simulink model "chaos_buck_CCM"  (R2021a)
settings: Solver=ode8  StartTime=0.0  StopTime=0.1  FixedStep=1e-6  RelTol=1e-3
model workspace (MAT data in the model file):
  C = Simulink.Parameter
  C.Value = [2.5e-05 2.51e-05 2.52e-05 2.53e-05 2.54e-05 2.55e-05 2.56e-05 2.57e-05 2.58e-05 2.59e-05 2.6e-05 2.61e-05 ... (351 elements, 1x351)]
  C.DataType = 'auto'
  C.Dimensions = [1 351]
  L = Simulink.Parameter
  L.Value = [0.01 0.0101 0.0102 0.0103 0.0104 0.0105 0.0106 0.0107 0.0108 0.0109 0.011 0.0111 0.0112 0.0113 0.0114 0.0115 0.0116 0.0117 0.0118 0.0119 0.012 0.0121 0.0122 0.0123 0.0124 0.0125 0.0126 0.0127 0.0128 0.0129 0.013 0.0131 0.0132 0.0133 0.0134 0.0135 0.0136 0.0137 0.0138 0.0139 0.014 0.0141 0.0142 0.0143 0.0144 0.0145 0.0146 0.0147 0.0148 0.0149 0.015 0.0151 0.0152 0.0153 0.0154 0.0155 0.0156 0.0157 0.0158 0.0159 0.016 0.0161 0.0162 0.0163 0.0164 0.0165 0.0166 0.0167 0.0168 0.0169 0.017 0.0171 0.0172 0.0173 0.0174 0.0175 0.0176 0.0177 0.0178 0.0179 0.018 0.0181 0.0182 0.0183 0.0184 0.0185 0.0186 0.0187 0.0188 0.0189 0.019 0.0191 0.0192 0.0193 0.0194 0.0195 0.0196 0.0197 0.0198 0.0199 0.02 0.0201 0.0202 0.0203 0.0204 0.0205 0.0206 0.0207 0.0208 0.0209 0.021 0.0211 0.0212 0.0213 0.0214 0.0215 0.0216 0.0217 0.0218 0.0219 0.022 0.0221 0.0222 0.0223 0.0224 0.0225 0.0226 0.0227 0.0228 0.0229 0.023 0.0231 0.0232 0.0233 0.0234 0.0235 0.0236 0.0237 0.0238 0.0239 0.024 0.0241 0.0242 0.0243 0.0244 0.0245 0.0246 0.0247 0.0248 0.0249 0.025]
  L.DataType = 'auto'
  L.Dimensions = [1 151]
  Vin = Simulink.Parameter
  Vin.Value = [20 20.1 20.2 20.3 20.4 20.5 20.6 20.7 20.8 20.9 21 21.1 21.2 21.3 21.4 21.5 21.6 21.7 21.8 21.9 22 22.1 22.2 22.3 22.4 22.5 22.6 22.7 22.8 22.9 23 23.1 23.2 23.3 23.4 23.5 23.6 23.7 23.8 23.9 24 24.1 24.2 24.3 24.4 24.5 24.6 24.7 24.8 24.9 25 25.1 25.2 25.3 25.4 25.5 25.6 25.7 25.8 25.9 26 26.1 26.2 26.3 26.4 26.5 26.6 26.7 26.8 26.9 27 27.1 27.2 27.3 27.4 27.5 27.6 27.7 27.8 27.9 28 28.1 28.2 28.3 28.4 28.5 28.6 28.7 28.8 28.9 29 29.1 29.2 29.3 29.4 29.5 29.6 29.7 29.8 29.9 30 30.1 30.2 30.3 30.4 30.5 30.6 30.7 30.8 30.9 31 31.1 31.2 31.3 31.4 31.5 31.6 31.7 31.8 31.9 32 32.1 32.2 32.3 32.4 32.5 32.6 32.7 32.8 32.9 33 33.1 33.2 33.3 33.4 33.5 33.6 33.7 33.8 33.9 34 34.1 34.2 34.3 34.4 34.5 34.6 34.7 34.8 34.9 35]
  Vin.DataType = 'auto'
  Vin.Dimensions = [1 151]
values from neighbouring files (symbols this model uses):
  Vin = 22    [CCM_iterative_mapping.m]    (also in DCM_iterative_mapping_bifur.m = 33)
libraries: simulink x1
settings Model: OrderedModelArguments=off  Creator=xiang zhang  LastModifiedBy=xiang zhang

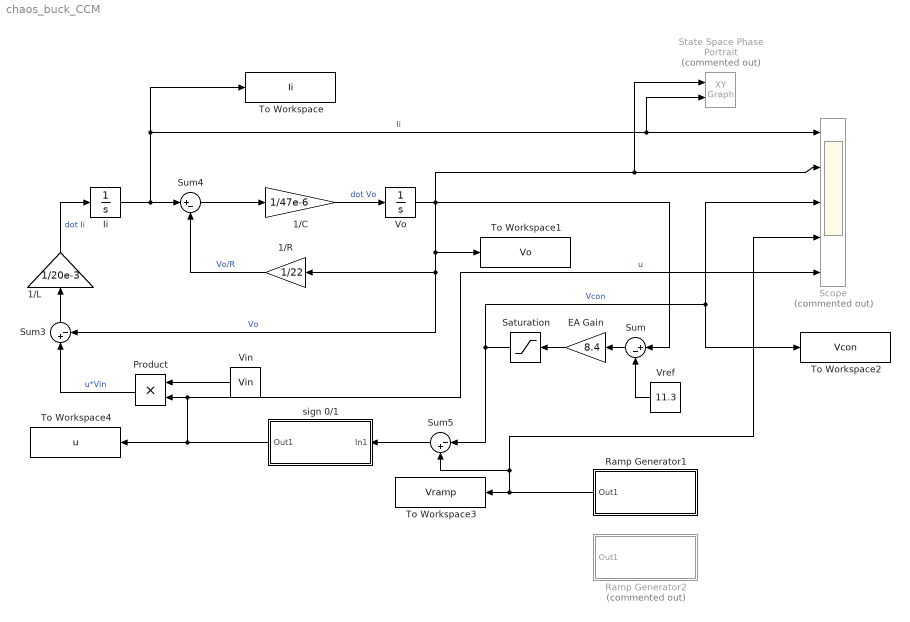
== system chaos_buck_CCM ==
  1/C : Gain  Gain=1/47e-6
  1/L : Gain  Gain=1/20e-3
  1/R : Gain  Gain=1/22
  EA Gain : Gain  Gain=8.4
  Ii : Integrator
  Product : Product
  Ramp Generator1 : Subsystem
  Ramp Generator2 : Subsystem  Commented=on
  Saturation : Saturate  UpperLimit=8.2  LowerLimit=3.8
  Scope : Scope  Commented=on  NumInputPorts=5
  State Space Phase Portrait : simulink/Sinks/XY Graph  Commented=on  xmin=10  xmax=14  ymin=-0.5  ymax=1.5  st=-1
  Sum : Sum  Inputs=|+-
  Sum3 : Sum  Inputs=|+-
  Sum4 : Sum  Inputs=|+-
  Sum5 : Sum  Inputs=|-+
  To Workspace : ToWorkspace  VariableName=Ii  SaveFormat=Timeseries  SampleTime=-1
  To Workspace1 : ToWorkspace  VariableName=Vo  SaveFormat=Timeseries  SampleTime=-1
  To Workspace2 : ToWorkspace  VariableName=Vcon  SaveFormat=Timeseries  SampleTime=-1
  To Workspace3 : ToWorkspace  VariableName=Vramp  SaveFormat=Timeseries  SampleTime=-1
  To Workspace4 : ToWorkspace  VariableName=u  SaveFormat=Timeseries  SampleTime=-1
  Vin : Constant  Value=Vin
  Vo : Integrator
  Vref : Constant  Value=11.3
  sign 0/1 : Subsystem
  wires:
  Vref/1 -> Sum/2
  Sum/1 -> EA Gain/1
  EA Gain/1 -> Saturation/1
  Sum5/1 -> sign 0/1/1(In1)
  Vin/1 -> Product/1
  Product/1 -> Sum3/1  "u*Vin"
  Sum3/1 -> 1/L/1
  1/L/1 -> Ii/1  "dot Ii"
  Ii/1 -> To Workspace/1, State Space Phase Portrait/2, Scope/1, Sum4/1  "Ii"
  Sum4/1 -> 1/C/1
  1/R/1 -> Sum4/2  "Vo/R"
  1/C/1 -> Vo/1  "dot Vo"
  Vo/1 -> Sum3/2, 1/R/1, To Workspace1/1, State Space Phase Portrait/1, Scope/2, Sum/1  "Vo"
  sign 0/1/1(Out1) -> Product/2, Scope/5, To Workspace4/1  "u"
  Saturation/1 -> To Workspace2/1, Scope/3, Sum5/1  "Vcon"
  Ramp Generator1/1(Out1) -> Scope/4, Sum5/2, To Workspace3/1

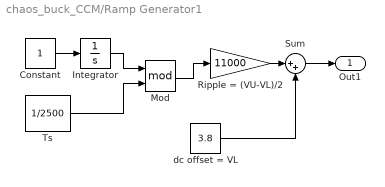
== system chaos_buck_CCM/Ramp Generator1 ==
  Constant : Constant
  Integrator : Integrator
  Mod : Math  Operator=mod  SaturateOnIntegerOverflow=on
  Ripple = (VU-VL)/2 : Gain  Gain=11000
  Sum : Sum  Inputs=|++
  Ts : Constant  Value=1/2500
  dc offset = VL : Constant  Value=3.8
  Out1 : Outport
  wires:
  Sum/1 -> Out1/1
  dc offset = VL/1 -> Sum/2
  Constant/1 -> Integrator/1
  Integrator/1 -> Mod/1
  Ripple = (VU-VL)/2/1 -> Sum/1
  Mod/1 -> Ripple = (VU-VL)/2/1
  Ts/1 -> Mod/2

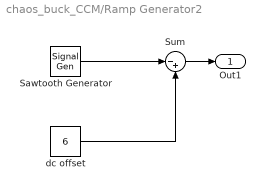
== system chaos_buck_CCM/Ramp Generator2 ==
  Sawtooth Generator : SignalGenerator  WaveForm=sawtooth  Amplitude=2.2  Frequency=2500  Units=rad/sec
  Sum : Sum  Inputs=|-+
  dc offset : Constant  Value=6
  Out1 : Outport
  wires:
  Sum/1 -> Out1/1
  Sawtooth Generator/1 -> Sum/1
  dc offset/1 -> Sum/2

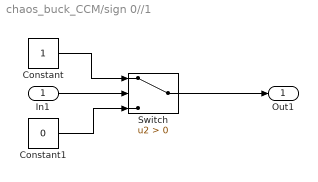
== system chaos_buck_CCM/sign 0//1 ==
  In1 : Inport
  Constant : Constant
  Constant1 : Constant  Value=0
  Switch : Switch  Criteria=u2 > Threshold
  Out1 : Outport
  wires:
  In1/1 -> Switch/2
  Switch/1 -> Out1/1
  Constant/1 -> Switch/1
  Constant1/1 -> Switch/3
